simulink model "dz4_longitudinal_ss"  (R2026a)
settings: Solver=ode45  StopTime=cfg.stop_time_s  MaxStep=1e-4  RelTol=1e-9  AbsTol=1e-11
model workspace (MAT data in the model file):
  A = [-0.0032239960127  2.48529585411  0  0  0; 0.0032239960127  -2.48529585411  0  1  0; 0  0  0  1  0; 0  -817.688207025  0  -6.68062624856  0; 470.139650123  0  0  0  0]
  B = [0.632544660979; -0.632544660979; 0; -957.29021238; 0]
  C = [1  0  0  0  0; 0  1  0  0  0; 0  0  1  0  0; 0  0  0  1  0; 0  0  0  0  1]
  D = [0; 0; 0; 0; 0]
  cfg.variant_id = 1
  cfg.g_mps2 = 9.81
  cfg.aircraft_type = "normal"
  cfg.control_sign = -1
  cfg.m = 44
  cfg.Iz = 13.46
  cfg.S = 0.022
  cfg.L = 1.88
  cfg.V = 476
  cfg.P = 8000
  cfg.rho = 1.13
  cfg.theta_deg = -9
  cfg.alpha_deg = 0.6
  cfg.theta_rad = -0.157079632679
  cfg.alpha_rad = 0.010471975512
  cfg.cy_alpha_per_deg = 0.273
  cfg.cy_delta_per_deg = 0.0821
  cfg.mz_alpha_per_deg = -0.03628
  cfg.mz_delta_per_deg = -0.042474
  cfg.cy_alpha = 15.6417478071
  cfg.cy_delta = 4.70398349802
  cfg.mz_alpha = -2.07869088073
  cfg.mz_delta = -2.43358093904
  cfg.mz_omega = -4.3
  cfg.delta_command_deg = 4
  cfg.delta_step_rad = -0.0698131700798
  cfg.step_time_s = 1
  cfg.stop_time_s = 9
settings Model: Creator=ievge  LastModifiedBy=ievge

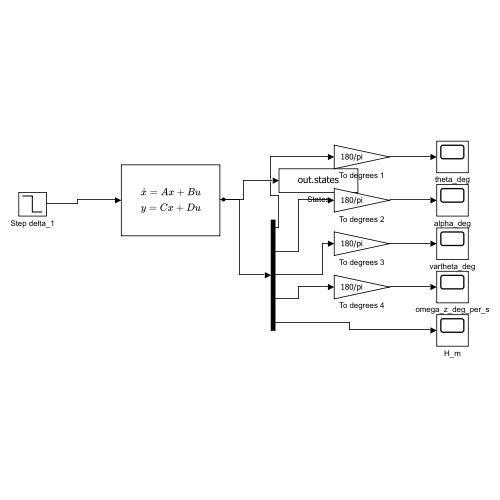
[thumbnail: Simulink's stored preview of the top-level diagram]
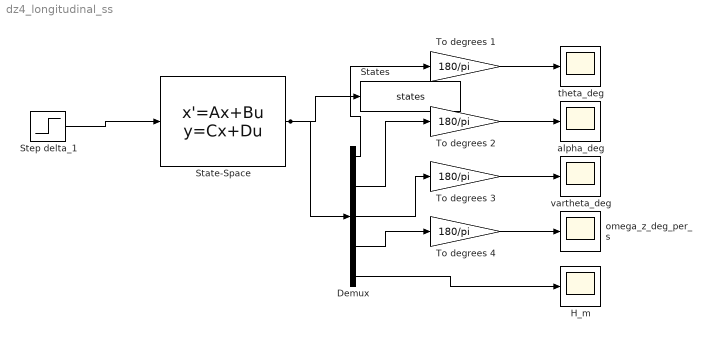
== system dz4_longitudinal_ss ==
  Demux : Demux  Outputs=5
  H_m : Scope
  State-Space : StateSpace  A=A  B=B  C=C  D=D  InitialCondition=zeros(5,1)
  States : ToWorkspace  VariableName=states  SaveFormat=Structure With Time  SampleTime=-1
  Step delta_1 : Step  Time=cfg.step_time_s  FinalValue=cfg.delta_step_rad  SampleTime=0
  To degrees {1..4} (4 alike) : Gain  Gain=180/pi
  alpha_deg : Scope
  omega_z_deg_per_s : Scope
  theta_deg : Scope
  vartheta_deg : Scope
  wires:
  Demux/1 -> To degrees 1/1
  To degrees 1/1 -> theta_deg/1
  Demux/2 -> To degrees 2/1
  To degrees 2/1 -> alpha_deg/1
  Demux/3 -> To degrees 3/1
  To degrees 3/1 -> vartheta_deg/1
  Demux/4 -> To degrees 4/1
  To degrees 4/1 -> omega_z_deg_per_s/1
  Demux/5 -> H_m/1
  Step delta_1/1 -> State-Space/1
  State-Space/1 -> States/1, Demux/1
